simulink model "ANN2"  (R2023a)
settings: Solver=VariableStepAuto  StartTime=0.0  StopTime=T_e  RelTol=1e-3
libraries: neural x50
(part 2 of 2)

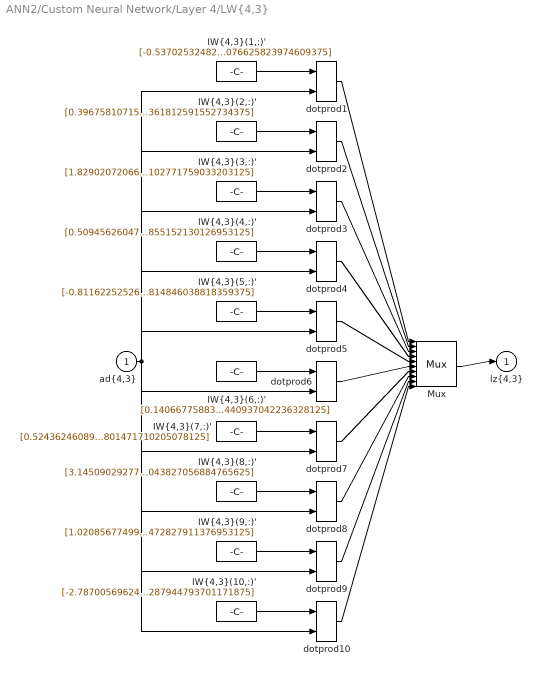
== system ANN2/Custom Neural Network/Layer 4/LW{4,3} ==
  "ad{4,3}" : Inport  PortDimensions=10
      mask Display: e = 0.06;c1 = [120 230 180]/255;c2 = ([120 230 180]+0)/(256+128);c3 = ([120 230 180]+128)/(256+128);patch([0 1 1 0],[0 0 1 1],c1);patch([0 1 1 1-e 1-e 0+e],[0 0 1 1-e 0+e 0+e],c2);patch([0 0 1 1-e 0+e 0+e],[0 1 1 1-e 1-e 0+e],c3);plot([0 1 1 0 0],[0 0 1 1 0]);
  "IW{4,3}(1,:)'" : Constant  Value=[-0.537025324828745542760088937939144670963287353515625;1.1446680784204037450990654178895056247711181640625;-0.1494718771280706681725547468886361457407474517822265625;0.5479329564740085256602242225199006497859954833984375;-1.669642114593291370994165845331735908985137939453125;-0.5625793961549316879455773232621140778064727783203125;-0.290840794289171922226699962266138754785060882568359375;0.392733785328576445738946176788886077702045440673828125;-0.1789140215041436221543591500449110753834247589111328125;-1.086491666232040298467609318322502076625823974609375]
      mask Display: e = 0.06;c1 = [120 150 230]/255;c2 = ([120 150 230]+0)/383;c3 = ([120 150 230]+128)/383;patch([0 1 1 0],[0 0 1 1],c1);patch([0 1 1 1-e 1-e 0+e],[0 0 1 1-e 0+e 0+e],c2);patch([0 0 1 1-e 0+e 0+e],[0 1 1 1-e 1-e 0+e],c3);plot([0 1 1 0 0],[0 0 1 1 0]);disp('weights');
  "IW{4,3}(10,:)'" : Constant  Value=[-2.787005696248002539761046136845834553241729736328125;0.355445992727688897527826838995679281651973724365234375;-3.332874567433335766253321708063594996929168701171875;-0.9149606460401908947233096114359796047210693359375;5.7559954570456710598591598682105541229248046875;-0.99078106892069339739492761509609408676624298095703125;0.5475894791811557471561400234350003302097320556640625;2.380184173476134645852653193287551403045654296875;3.959959795795794601502848308882676064968109130859375;-2.121256431157334088055677057127468287944793701171875]
      mask Display: e = 0.06;c1 = [120 150 230]/255;c2 = ([120 150 230]+0)/383;c3 = ([120 150 230]+128)/383;patch([0 1 1 0],[0 0 1 1],c1);patch([0 1 1 1-e 1-e 0+e],[0 0 1 1-e 0+e 0+e],c2);patch([0 0 1 1-e 0+e 0+e],[0 1 1 1-e 1-e 0+e],c3);plot([0 1 1 0 0],[0 0 1 1 0]);disp('weights');
  "IW{4,3}(2,:)'" : Constant  Value=[0.396758107155528672027600123328738845884799957275390625;-0.7982495408802090519628791298600845038890838623046875;1.09104310519050518024641860392875969409942626953125;-0.71608447177029777019896528145181946456432342529296875;-1.552094486706580678259115302353166043758392333984375;-3.48288477851992350764476213953457772731781005859375;1.168858832263365510328867458156310021877288818359375;3.407206318151043245023856798070482909679412841796875;1.8423773332868151886287932939012534916400909423828125;-1.014961278667806165998399592353962361812591552734375]
      mask Display: e = 0.06;c1 = [120 150 230]/255;c2 = ([120 150 230]+0)/383;c3 = ([120 150 230]+128)/383;patch([0 1 1 0],[0 0 1 1],c1);patch([0 1 1 1-e 1-e 0+e],[0 0 1 1-e 0+e 0+e],c2);patch([0 0 1 1-e 0+e 0+e],[0 1 1 1-e 1-e 0+e],c3);plot([0 1 1 0 0],[0 0 1 1 0]);disp('weights');
  "IW{4,3}(3,:)'" : Constant  Value=[1.8290207206670807682513668623869307339191436767578125;0.8943810142493828774234998491010628640651702880859375;1.056079773271772825893322078627534210681915283203125;0.1880359070482093830634084952180273830890655517578125;-1.3709952682832400316925713923410512506961822509765625;-1.66389250084688367081753312959335744380950927734375;-0.7960652672681340913385383828426711261272430419921875;0.01201426242866930095554156565640369080938398838043212890625;2.1321803493174211752148039522580802440643310546875;-2.89388260379740547278970552724786102771759033203125]
      mask Display: e = 0.06;c1 = [120 150 230]/255;c2 = ([120 150 230]+0)/383;c3 = ([120 150 230]+128)/383;patch([0 1 1 0],[0 0 1 1],c1);patch([0 1 1 1-e 1-e 0+e],[0 0 1 1-e 0+e 0+e],c2);patch([0 0 1 1-e 0+e 0+e],[0 1 1 1-e 1-e 0+e],c3);plot([0 1 1 0 0],[0 0 1 1 0]);disp('weights');
  "IW{4,3}(4,:)'" : Constant  Value=[0.5094562604743864131506825287942774593830108642578125;-0.1271628532297165159459240157957538031041622161865234375;-0.0167441158582526637699228189148925594054162502288818359375;-0.68414310749160434088622650961042381823062896728515625;-0.126156232581473404241734215247561223804950714111328125;0.60413901637336253624965820563375018537044525146484375;0.3846873784056101808204175540595315396785736083984375;0.24254796061830508069334655374404974281787872314453125;-0.224400612886833439318934324546717107295989990234375;1.0503482574470812682676523763802833855152130126953125]
      mask Display: e = 0.06;c1 = [120 150 230]/255;c2 = ([120 150 230]+0)/383;c3 = ([120 150 230]+128)/383;patch([0 1 1 0],[0 0 1 1],c1);patch([0 1 1 1-e 1-e 0+e],[0 0 1 1-e 0+e 0+e],c2);patch([0 0 1 1-e 0+e 0+e],[0 1 1 1-e 1-e 0+e],c3);plot([0 1 1 0 0],[0 0 1 1 0]);disp('weights');
  "IW{4,3}(5,:)'" : Constant  Value=[-0.811622525269869665720534612773917615413665771484375;-1.4106025169422549137010491904220543801784515380859375;-0.0183018997177856433677956005112719140015542507171630859375;3.89309146846569120725689572282135486602783203125;-1.50908859273326800831682703574188053607940673828125;1.46141531167657579004526269272901117801666259765625;-0.150275881711567638188142836952465586364269256591796875;1.6297483708125570789349012557067908346652984619140625;-1.5428389049328325999255184797220863401889801025390625;-0.63185372991077881632548951529315672814846038818359375]
      mask Display: e = 0.06;c1 = [120 150 230]/255;c2 = ([120 150 230]+0)/383;c3 = ([120 150 230]+128)/383;patch([0 1 1 0],[0 0 1 1],c1);patch([0 1 1 1-e 1-e 0+e],[0 0 1 1-e 0+e 0+e],c2);patch([0 0 1 1-e 0+e 0+e],[0 1 1 1-e 1-e 0+e],c3);plot([0 1 1 0 0],[0 0 1 1 0]);disp('weights');
  "IW{4,3}(6,:)'" : Constant  Value=[0.140667758835533784900206910606357268989086151123046875;-0.33082048644864225916961686380091123282909393310546875;2.8943147000219067166426611947827041149139404296875;0.46843943618673378193051348716835491359233856201171875;1.0496618859311921401200606851489283144474029541015625;-4.1579973534433047888114742818288505077362060546875;0.5783757929523909435687301083817146718502044677734375;1.92080277540615984577243580133654177188873291015625;-1.0833641680698453679809745153761468827724456787109375;-2.416592138388740096388573874719440937042236328125]
      mask Display: e = 0.06;c1 = [120 150 230]/255;c2 = ([120 150 230]+0)/383;c3 = ([120 150 230]+128)/383;patch([0 1 1 0],[0 0 1 1],c1);patch([0 1 1 1-e 1-e 0+e],[0 0 1 1-e 0+e 0+e],c2);patch([0 0 1 1-e 0+e 0+e],[0 1 1 1-e 1-e 0+e],c3);plot([0 1 1 0 0],[0 0 1 1 0]);disp('weights');
  "IW{4,3}(7,:)'" : Constant  Value=[0.52436246089386429058976091255317442119121551513671875;2.62726665038294893150805364712141454219818115234375;0.27213786631926628611921614719904027879238128662109375;0.173338632167647166415491710722562856972217559814453125;-0.49428272542603257644344694199389778077602386474609375;-0.5905815273629093642426823862479068338871002197265625;-1.665709768844600535686595321749337017536163330078125;2.151571280856003465231651716749183833599090576171875;-0.99245428187803408359712875608238391578197479248046875;-0.8722814140498649226884708696161396801471710205078125]
      mask Display: e = 0.06;c1 = [120 150 230]/255;c2 = ([120 150 230]+0)/383;c3 = ([120 150 230]+128)/383;patch([0 1 1 0],[0 0 1 1],c1);patch([0 1 1 1-e 1-e 0+e],[0 0 1 1-e 0+e 0+e],c2);patch([0 0 1 1-e 0+e 0+e],[0 1 1 1-e 1-e 0+e],c3);plot([0 1 1 0 0],[0 0 1 1 0]);disp('weights');
  "IW{4,3}(8,:)'" : Constant  Value=[3.145090292773045081986538207274861633777618408203125;-3.86518867354375483813555547385476529598236083984375;2.84019382107351692212660054792650043964385986328125;1.55926295353270916166366077959537506103515625;0.039683951825970710525215423558620386756956577301025390625;-5.84857444485736976957923616282641887664794921875;0.41805408872401728093137762698461301624774932861328125;0.9154501482653378818810097072855569422245025634765625;2.83146209099063828062980974209494888782501220703125;-2.81443369574421442536049653426744043827056884765625]
      mask Display: e = 0.06;c1 = [120 150 230]/255;c2 = ([120 150 230]+0)/383;c3 = ([120 150 230]+128)/383;patch([0 1 1 0],[0 0 1 1],c1);patch([0 1 1 1-e 1-e 0+e],[0 0 1 1-e 0+e 0+e],c2);patch([0 0 1 1-e 0+e 0+e],[0 1 1 1-e 1-e 0+e],c3);plot([0 1 1 0 0],[0 0 1 1 0]);disp('weights');
  "IW{4,3}(9,:)'" : Constant  Value=[1.0208567749915384847980703852954320609569549560546875;1.8582832947571130688402263331227004528045654296875;-4.74241761861468802408126066438853740692138671875;3.34339941696541931293040761374868452548980712890625;-4.3852798112980195810450823046267032623291015625;0.96443219351488529422766760035301558673381805419921875;-0.11001563040819332950359665801443043164908885955810546875;4.5826383567559556553305810666643083095550537109375;-2.265268244805841657552036849665455520153045654296875;-2.904982027231259866795198831823654472827911376953125]
      mask Display: e = 0.06;c1 = [120 150 230]/255;c2 = ([120 150 230]+0)/383;c3 = ([120 150 230]+128)/383;patch([0 1 1 0],[0 0 1 1],c1);patch([0 1 1 1-e 1-e 0+e],[0 0 1 1-e 0+e 0+e],c2);patch([0 0 1 1-e 0+e 0+e],[0 1 1 1-e 1-e 0+e],c3);plot([0 1 1 0 0],[0 0 1 1 0]);disp('weights');
  Mux : Mux  Inputs=10
      mask Display: e = 0.06;c1 = [120 150 230]/255;c2 = ([120 150 230]+0)/383;c3 = ([120 150 230]+128)/383;patch([0 1 1 0],[0 0 1 1],c1);patch([0 1 1 1-e 1-e 0+e],[0 0 1 1-e 0+e 0+e],c2);patch([0 0 1 1-e 0+e 0+e],[0 1 1 1-e 1-e 0+e],c3);plot([0 1 1 0 0],[0 0 1 1 0]);disp('Mux');
  dotprod{1..10} (10 alike) : neural/Weight Functions/dotprod
  "lz{4,3}" : Outport
      mask Display: e = 0.06;c1 = [120 230 180]/255;c2 = ([120 230 180]+0)/(256+128);c3 = ([120 230 180]+128)/(256+128);patch([0 1 1 0],[0 0 1 1],c1);patch([0 1 1 1-e 1-e 0+e],[0 0 1 1-e 0+e 0+e],c2);patch([0 0 1 1-e 0+e 0+e],[0 1 1 1-e 1-e 0+e],c3);plot([0 1 1 0 0],[0 0 1 1 0]);
  wires:
  "IW{4,3}(1,:)'"/1 -> dotprod1/1
  "ad{4,3}"/1 -> dotprod1/2, dotprod2/2, dotprod3/2, dotprod4/2, dotprod5/2, dotprod6/2, dotprod7/2, dotprod8/2, dotprod9/2, dotprod10/2
  dotprod1/1 -> Mux/1
  "IW{4,3}(2,:)'"/1 -> dotprod2/1
  dotprod2/1 -> Mux/2
  "IW{4,3}(3,:)'"/1 -> dotprod3/1
  dotprod3/1 -> Mux/3
  "IW{4,3}(4,:)'"/1 -> dotprod4/1
  dotprod4/1 -> Mux/4
  "IW{4,3}(5,:)'"/1 -> dotprod5/1
  dotprod5/1 -> Mux/5
  "IW{4,3}(6,:)'"/1 -> dotprod6/1
  dotprod6/1 -> Mux/6
  "IW{4,3}(7,:)'"/1 -> dotprod7/1
  dotprod7/1 -> Mux/7
  "IW{4,3}(8,:)'"/1 -> dotprod8/1
  dotprod8/1 -> Mux/8
  "IW{4,3}(9,:)'"/1 -> dotprod9/1
  dotprod9/1 -> Mux/9
  "IW{4,3}(10,:)'"/1 -> dotprod10/1
  dotprod10/1 -> Mux/10
  Mux/1 -> "lz{4,3}"/1

== system ANN2/Custom Neural Network/Layer 5/Delays 1 ==
  "p{5}" : Inport  PortDimensions=10
      mask Display: e = 0.06;c1 = [120 230 180]/255;c2 = ([120 230 180]+0)/(256+128);c3 = ([120 230 180]+128)/(256+128);patch([0 1 1 0],[0 0 1 1],c1);patch([0 1 1 1-e 1-e 0+e],[0 0 1 1-e 0+e 0+e],c2);patch([0 0 1 1-e 0+e 0+e],[0 1 1 1-e 1-e 0+e],c3);plot([0 1 1 0 0],[0 0 1 1 0]);
  mux : Mux  Inputs=1
      mask Display: e = 0.06;c1 = [120 150 230]/255;c2 = ([120 150 230]+0)/383;c3 = ([120 150 230]+128)/383;patch([0 1 1 0],[0 0 1 1],c1);patch([0 1 1 1-e 1-e 0+e],[0 0 1 1-e 0+e 0+e],c2);patch([0 0 1 1-e 0+e 0+e],[0 1 1 1-e 1-e 0+e],c3);plot([0 1 1 0 0],[0 0 1 1 0]);disp('Mux')
  "pd{5,4}" : Outport
      mask Display: e = 0.06;c1 = [120 230 180]/255;c2 = ([120 230 180]+0)/(256+128);c3 = ([120 230 180]+128)/(256+128);patch([0 1 1 0],[0 0 1 1],c1);patch([0 1 1 1-e 1-e 0+e],[0 0 1 1-e 0+e 0+e],c2);patch([0 0 1 1-e 0+e 0+e],[0 1 1 1-e 1-e 0+e],c3);plot([0 1 1 0 0],[0 0 1 1 0]);
  wires:
  "p{5}"/1 -> mux/1
  mux/1 -> "pd{5,4}"/1

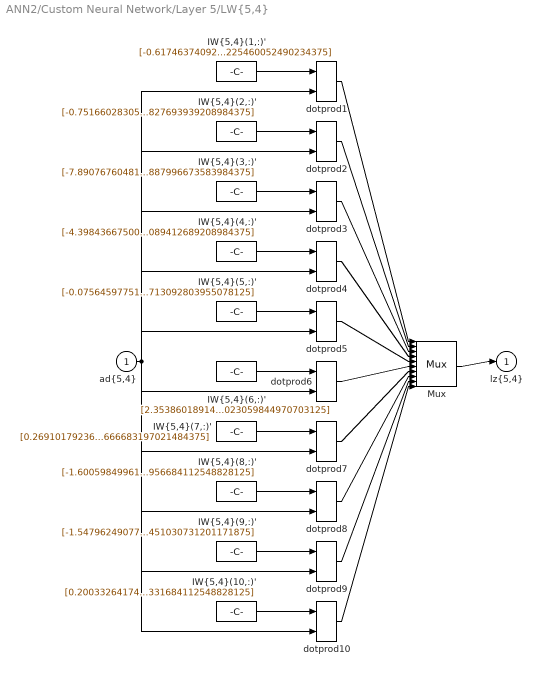
== system ANN2/Custom Neural Network/Layer 5/LW{5,4} ==
  "ad{5,4}" : Inport  PortDimensions=10
      mask Display: e = 0.06;c1 = [120 230 180]/255;c2 = ([120 230 180]+0)/(256+128);c3 = ([120 230 180]+128)/(256+128);patch([0 1 1 0],[0 0 1 1],c1);patch([0 1 1 1-e 1-e 0+e],[0 0 1 1-e 0+e 0+e],c2);patch([0 0 1 1-e 0+e 0+e],[0 1 1 1-e 1-e 0+e],c3);plot([0 1 1 0 0],[0 0 1 1 0]);
  "IW{5,4}(1,:)'" : Constant  Value=[-0.61746374092532685384782098481082357466220855712890625;-0.74954619667786193115688320176559500396251678466796875;1.0833816431203151520179517319775186479091644287109375;1.7369431809461681748274486380978487432003021240234375;1.553732116597537515900739890639670193195343017578125;1.2894407873928981356215217601857148110866546630859375;-0.942531357935733726804983234615065157413482666015625;0.32674094499821182413512588027515448629856109619140625;-2.13633767789866624298156239092350006103515625;0.94964139675599434919917030128999613225460052490234375]
      mask Display: e = 0.06;c1 = [120 150 230]/255;c2 = ([120 150 230]+0)/383;c3 = ([120 150 230]+128)/383;patch([0 1 1 0],[0 0 1 1],c1);patch([0 1 1 1-e 1-e 0+e],[0 0 1 1-e 0+e 0+e],c2);patch([0 0 1 1-e 0+e 0+e],[0 1 1 1-e 1-e 0+e],c3);plot([0 1 1 0 0],[0 0 1 1 0]);disp('weights');
  "IW{5,4}(10,:)'" : Constant  Value=[0.2003326417468528630738688889323384501039981842041015625;-1.4035509099787955022975438623689115047454833984375;0.758724425225181686727182750473730266094207763671875;8.2265308932463607760610102559439837932586669921875;2.292982209538020565986471410724334418773651123046875;-0.5055975969964006111467824666760861873626708984375;0.1590020765484128906219751797834760509431362152099609375;2.422091846343718213319107235292904078960418701171875;4.02884240771798918245849563390947878360748291015625;-0.7688031110806108348043608202715404331684112548828125]
      mask Display: e = 0.06;c1 = [120 150 230]/255;c2 = ([120 150 230]+0)/383;c3 = ([120 150 230]+128)/383;patch([0 1 1 0],[0 0 1 1],c1);patch([0 1 1 1-e 1-e 0+e],[0 0 1 1-e 0+e 0+e],c2);patch([0 0 1 1-e 0+e 0+e],[0 1 1 1-e 1-e 0+e],c3);plot([0 1 1 0 0],[0 0 1 1 0]);disp('weights');
  "IW{5,4}(2,:)'" : Constant  Value=[-0.7516602830507712607044368269271217286586761474609375;1.6918604850429763697405860511935316026210784912109375;1.4564132621388503618931054006679914891719818115234375;-0.14240940879210939318255668695201165974140167236328125;0.50952281694995760208399815383017994463443756103515625;2.712135429031558242485289156320504844188690185546875;-4.98058075447596593221533112227916717529296875;-1.48008169270694889263495497289113700389862060546875;4.8035604982567985388186571071855723857879638671875;5.26519168037761886580483405850827693939208984375]
      mask Display: e = 0.06;c1 = [120 150 230]/255;c2 = ([120 150 230]+0)/383;c3 = ([120 150 230]+128)/383;patch([0 1 1 0],[0 0 1 1],c1);patch([0 1 1 1-e 1-e 0+e],[0 0 1 1-e 0+e 0+e],c2);patch([0 0 1 1-e 0+e 0+e],[0 1 1 1-e 1-e 0+e],c3);plot([0 1 1 0 0],[0 0 1 1 0]);disp('weights');
  "IW{5,4}(3,:)'" : Constant  Value=[-7.8907676048188033490760062704794108867645263671875;0.981295218285413994863120024092495441436767578125;6.12998698487287274616619470180012285709381103515625;1.58187690612738851569929465767927467823028564453125;-0.1674823712869970837591182544201728887856006622314453125;5.29070079873718679408511889050714671611785888671875;-9.5234000430462497632788654300384223461151123046875;0.043157361994706246177688768739244551397860050201416015625;-2.451603015838451415930876464699395000934600830078125;-2.161503528686553377013979115872643887996673583984375]
      mask Display: e = 0.06;c1 = [120 150 230]/255;c2 = ([120 150 230]+0)/383;c3 = ([120 150 230]+128)/383;patch([0 1 1 0],[0 0 1 1],c1);patch([0 1 1 1-e 1-e 0+e],[0 0 1 1-e 0+e 0+e],c2);patch([0 0 1 1-e 0+e 0+e],[0 1 1 1-e 1-e 0+e],c3);plot([0 1 1 0 0],[0 0 1 1 0]);disp('weights');
  "IW{5,4}(4,:)'" : Constant  Value=[-4.39843667500335033793135153246112167835235595703125;0.75697252719984031710254157587769441306591033935546875;0.6713197339275713826367564251995645463466644287109375;-5.19984551356537405553126518498174846172332763671875;-0.005200057200189901231157652006231728591956198215484619140625;-0.8542551830036788640398981442558579146862030029296875;-3.67183975580720112219523798557929694652557373046875;-0.09340205117695034309210910805632011033594608306884765625;-2.601031547024164058967699020286090672016143798828125;0.29690667739951892567518143550842069089412689208984375]
      mask Display: e = 0.06;c1 = [120 150 230]/255;c2 = ([120 150 230]+0)/383;c3 = ([120 150 230]+128)/383;patch([0 1 1 0],[0 0 1 1],c1);patch([0 1 1 1-e 1-e 0+e],[0 0 1 1-e 0+e 0+e],c2);patch([0 0 1 1-e 0+e 0+e],[0 1 1 1-e 1-e 0+e],c3);plot([0 1 1 0 0],[0 0 1 1 0]);disp('weights');
  "IW{5,4}(5,:)'" : Constant  Value=[-0.07564597751843739337207495054826722480356693267822265625;-0.351126506377010982884456780084292404353618621826171875;1.3504338598524092684982633727486245334148406982421875;4.895111913238050505015053204260766506195068359375;2.450088651779480652947995622525922954082489013671875;1.933133653314374367226946560549549758434295654296875;-0.30691598672401398939513228469877503812313079833984375;2.080944975471171520808866262086667120456695556640625;-4.2680049412036371592193972901441156864166259765625;0.8228630166311738936002484479104168713092803955078125]
      mask Display: e = 0.06;c1 = [120 150 230]/255;c2 = ([120 150 230]+0)/383;c3 = ([120 150 230]+128)/383;patch([0 1 1 0],[0 0 1 1],c1);patch([0 1 1 1-e 1-e 0+e],[0 0 1 1-e 0+e 0+e],c2);patch([0 0 1 1-e 0+e 0+e],[0 1 1 1-e 1-e 0+e],c3);plot([0 1 1 0 0],[0 0 1 1 0]);disp('weights');
  "IW{5,4}(6,:)'" : Constant  Value=[2.353860189142553682728475905605591833591461181640625;0.9891004184910467955660351435653865337371826171875;0.487783761163201656785304294317029416561126708984375;-0.62813387874629900142764427073416300117969512939453125;-0.8714125912064367707188239364768378436565399169921875;-0.70410209563019232614777820344897918403148651123046875;-5.005847642266104458030895330011844635009765625;-0.226240064872049229105499534853151999413967132568359375;-3.4273271244920540112843809765763580799102783203125;1.916044779447613866096844503772445023059844970703125]
      mask Display: e = 0.06;c1 = [120 150 230]/255;c2 = ([120 150 230]+0)/383;c3 = ([120 150 230]+128)/383;patch([0 1 1 0],[0 0 1 1],c1);patch([0 1 1 1-e 1-e 0+e],[0 0 1 1-e 0+e 0+e],c2);patch([0 0 1 1-e 0+e 0+e],[0 1 1 1-e 1-e 0+e],c3);plot([0 1 1 0 0],[0 0 1 1 0]);disp('weights');
  "IW{5,4}(7,:)'" : Constant  Value=[0.269101792362137326453108698842697776854038238525390625;-1.3775123335482424291598135823733173310756683349609375;-3.314642270519360778280315571464598178863525390625;-1.2521397119053740976113431315752677619457244873046875;-4.9149350086204197651795766432769596576690673828125;-1.4409662719510649697696180737693794071674346923828125;0.60080378360446473617884066698024980723857879638671875;-0.69243558734772714391425552094005979597568511962890625;1.63020317845029705239312534104101359844207763671875;-0.7232648889974784278678043847321532666683197021484375]
      mask Display: e = 0.06;c1 = [120 150 230]/255;c2 = ([120 150 230]+0)/383;c3 = ([120 150 230]+128)/383;patch([0 1 1 0],[0 0 1 1],c1);patch([0 1 1 1-e 1-e 0+e],[0 0 1 1-e 0+e 0+e],c2);patch([0 0 1 1-e 0+e 0+e],[0 1 1 1-e 1-e 0+e],c3);plot([0 1 1 0 0],[0 0 1 1 0]);disp('weights');
  "IW{5,4}(8,:)'" : Constant  Value=[-1.6005984996132653908063048220355994999408721923828125;7.69142008725226045129375052056275308132171630859375;4.9870910262057055462037169490940868854522705078125;0.8056805537796798422078836665605194866657257080078125;7.60928821046500303282300592400133609771728515625;-2.74403381329962403611943955183960497379302978515625;-6.97512021113505564784418311319313943386077880859375;-1.5490438227356080336249988249619491398334503173828125;-7.419676016823661512944454443641006946563720703125;-0.84030296411506200104923891558428294956684112548828125]
      mask Display: e = 0.06;c1 = [120 150 230]/255;c2 = ([120 150 230]+0)/383;c3 = ([120 150 230]+128)/383;patch([0 1 1 0],[0 0 1 1],c1);patch([0 1 1 1-e 1-e 0+e],[0 0 1 1-e 0+e 0+e],c2);patch([0 0 1 1-e 0+e 0+e],[0 1 1 1-e 1-e 0+e],c3);plot([0 1 1 0 0],[0 0 1 1 0]);disp('weights');
  "IW{5,4}(9,:)'" : Constant  Value=[-1.5479624907750169082731872549629770219326019287109375;2.1454711850043661769404934602789580821990966796875;1.9222001346013255496103511177352629601955413818359375;0.17478859229319498869159588139154948294162750244140625;1.4730767216919848916489854673272930085659027099609375;-2.370608031768721257748211428406648337841033935546875;-0.6410368908050327885206343125901184976100921630859375;0.1555018189508294568224044951421092264354228973388671875;-2.9864606407143323707487070350907742977142333984375;-2.058350948652772682834211082081310451030731201171875]
      mask Display: e = 0.06;c1 = [120 150 230]/255;c2 = ([120 150 230]+0)/383;c3 = ([120 150 230]+128)/383;patch([0 1 1 0],[0 0 1 1],c1);patch([0 1 1 1-e 1-e 0+e],[0 0 1 1-e 0+e 0+e],c2);patch([0 0 1 1-e 0+e 0+e],[0 1 1 1-e 1-e 0+e],c3);plot([0 1 1 0 0],[0 0 1 1 0]);disp('weights');
  Mux : Mux  Inputs=10
      mask Display: e = 0.06;c1 = [120 150 230]/255;c2 = ([120 150 230]+0)/383;c3 = ([120 150 230]+128)/383;patch([0 1 1 0],[0 0 1 1],c1);patch([0 1 1 1-e 1-e 0+e],[0 0 1 1-e 0+e 0+e],c2);patch([0 0 1 1-e 0+e 0+e],[0 1 1 1-e 1-e 0+e],c3);plot([0 1 1 0 0],[0 0 1 1 0]);disp('Mux');
  dotprod{1..10} (10 alike) : neural/Weight Functions/dotprod
  "lz{5,4}" : Outport
      mask Display: e = 0.06;c1 = [120 230 180]/255;c2 = ([120 230 180]+0)/(256+128);c3 = ([120 230 180]+128)/(256+128);patch([0 1 1 0],[0 0 1 1],c1);patch([0 1 1 1-e 1-e 0+e],[0 0 1 1-e 0+e 0+e],c2);patch([0 0 1 1-e 0+e 0+e],[0 1 1 1-e 1-e 0+e],c3);plot([0 1 1 0 0],[0 0 1 1 0]);
  wires:
  "IW{5,4}(1,:)'"/1 -> dotprod1/1
  "ad{5,4}"/1 -> dotprod1/2, dotprod2/2, dotprod3/2, dotprod4/2, dotprod5/2, dotprod6/2, dotprod7/2, dotprod8/2, dotprod9/2, dotprod10/2
  dotprod1/1 -> Mux/1
  "IW{5,4}(2,:)'"/1 -> dotprod2/1
  dotprod2/1 -> Mux/2
  "IW{5,4}(3,:)'"/1 -> dotprod3/1
  dotprod3/1 -> Mux/3
  "IW{5,4}(4,:)'"/1 -> dotprod4/1
  dotprod4/1 -> Mux/4
  "IW{5,4}(5,:)'"/1 -> dotprod5/1
  dotprod5/1 -> Mux/5
  "IW{5,4}(6,:)'"/1 -> dotprod6/1
  dotprod6/1 -> Mux/6
  "IW{5,4}(7,:)'"/1 -> dotprod7/1
  dotprod7/1 -> Mux/7
  "IW{5,4}(8,:)'"/1 -> dotprod8/1
  dotprod8/1 -> Mux/8
  "IW{5,4}(9,:)'"/1 -> dotprod9/1
  dotprod9/1 -> Mux/9
  "IW{5,4}(10,:)'"/1 -> dotprod10/1
  dotprod10/1 -> Mux/10
  Mux/1 -> "lz{5,4}"/1

== system ANN2/Custom Neural Network/Layer 6/Delays 1 ==
  "p{6}" : Inport  PortDimensions=10
      mask Display: e = 0.06;c1 = [120 230 180]/255;c2 = ([120 230 180]+0)/(256+128);c3 = ([120 230 180]+128)/(256+128);patch([0 1 1 0],[0 0 1 1],c1);patch([0 1 1 1-e 1-e 0+e],[0 0 1 1-e 0+e 0+e],c2);patch([0 0 1 1-e 0+e 0+e],[0 1 1 1-e 1-e 0+e],c3);plot([0 1 1 0 0],[0 0 1 1 0]);
  mux : Mux  Inputs=1
      mask Display: e = 0.06;c1 = [120 150 230]/255;c2 = ([120 150 230]+0)/383;c3 = ([120 150 230]+128)/383;patch([0 1 1 0],[0 0 1 1],c1);patch([0 1 1 1-e 1-e 0+e],[0 0 1 1-e 0+e 0+e],c2);patch([0 0 1 1-e 0+e 0+e],[0 1 1 1-e 1-e 0+e],c3);plot([0 1 1 0 0],[0 0 1 1 0]);disp('Mux')
  "pd{6,5}" : Outport
      mask Display: e = 0.06;c1 = [120 230 180]/255;c2 = ([120 230 180]+0)/(256+128);c3 = ([120 230 180]+128)/(256+128);patch([0 1 1 0],[0 0 1 1],c1);patch([0 1 1 1-e 1-e 0+e],[0 0 1 1-e 0+e 0+e],c2);patch([0 0 1 1-e 0+e 0+e],[0 1 1 1-e 1-e 0+e],c3);plot([0 1 1 0 0],[0 0 1 1 0]);
  wires:
  "p{6}"/1 -> mux/1
  mux/1 -> "pd{6,5}"/1

== system ANN2/Custom Neural Network/Layer 6/LW{6,5} ==
  "ad{6,5}" : Inport  PortDimensions=10
      mask Display: e = 0.06;c1 = [120 230 180]/255;c2 = ([120 230 180]+0)/(256+128);c3 = ([120 230 180]+128)/(256+128);patch([0 1 1 0],[0 0 1 1],c1);patch([0 1 1 1-e 1-e 0+e],[0 0 1 1-e 0+e 0+e],c2);patch([0 0 1 1-e 0+e 0+e],[0 1 1 1-e 1-e 0+e],c3);plot([0 1 1 0 0],[0 0 1 1 0]);
  "IW{6,5}(1,:)'" : Constant  Value=[-1.7192297081165570649119445079122669994831085205078125;-0.35154526642192396312935898095020093023777008056640625;-1.4972770635967218577633275344851426780223846435546875;2.683712230655154851177712771459482610225677490234375;1.297656826401526242165118674165569245815277099609375;-2.24777978906358821831190653028897941112518310546875;-0.4769537579309093278112641201005317270755767822265625;0.494934633130672485545886729596531949937343597412109375;-0.81803531673359231035647098906338214874267578125;-1.45907223536778918315803821315057575702667236328125]
      mask Display: e = 0.06;c1 = [120 150 230]/255;c2 = ([120 150 230]+0)/383;c3 = ([120 150 230]+128)/383;patch([0 1 1 0],[0 0 1 1],c1);patch([0 1 1 1-e 1-e 0+e],[0 0 1 1-e 0+e 0+e],c2);patch([0 0 1 1-e 0+e 0+e],[0 1 1 1-e 1-e 0+e],c3);plot([0 1 1 0 0],[0 0 1 1 0]);disp('weights');
  Mux : Mux  Inputs=1
      mask Display: e = 0.06;c1 = [120 150 230]/255;c2 = ([120 150 230]+0)/383;c3 = ([120 150 230]+128)/383;patch([0 1 1 0],[0 0 1 1],c1);patch([0 1 1 1-e 1-e 0+e],[0 0 1 1-e 0+e 0+e],c2);patch([0 0 1 1-e 0+e 0+e],[0 1 1 1-e 1-e 0+e],c3);plot([0 1 1 0 0],[0 0 1 1 0]);disp('Mux');
  dotprod1 : neural/Weight Functions/dotprod
  "lz{6,5}" : Outport
      mask Display: e = 0.06;c1 = [120 230 180]/255;c2 = ([120 230 180]+0)/(256+128);c3 = ([120 230 180]+128)/(256+128);patch([0 1 1 0],[0 0 1 1],c1);patch([0 1 1 1-e 1-e 0+e],[0 0 1 1-e 0+e 0+e],c2);patch([0 0 1 1-e 0+e 0+e],[0 1 1 1-e 1-e 0+e],c3);plot([0 1 1 0 0],[0 0 1 1 0]);
  wires:
  "IW{6,5}(1,:)'"/1 -> dotprod1/1
  "ad{6,5}"/1 -> dotprod1/2
  dotprod1/1 -> Mux/1
  Mux/1 -> "lz{6,5}"/1

== matlab function ANN2/MATLAB Function ==
  data: u input; y output; v input; w input
function y = fcn(u,v,w)


all=[u;v;w];

y = all;
